simulink model "Simulacion_stepper_2024a"  (R2024a)
settings: Solver=ode4  StartTime=0.0  StopTime=Time_simulation  FixedStep=1/frecuency_simulation  RelTol=1e-3
InitFcn:
  | %%InitFcn();
StopFcn:
  | %%FinishFcn
model workspace (MAT data in the model file):
  Ts_stepper = 0.001
values from neighbouring files (symbols this model uses):
  B = motor_params.B_internal    [bode.m]    (also in current_observer.m = 0.0005; discretizacion.m = [ 1/L, 0; ekf_4_estados.m = params.B; obs_ctrl_back_emf_ext.m = [1/L 0)
  B0 = 3*wn_w - BJ_hat    [Barrido_B.m]    (also in Barrido_J.m; InitFcn.m = 449.962302294)
  B1 = 3*wn_w^2 - B0*BJ_hat    [Barrido_B.m]    (also in Barrido_J.m; InitFcn.m = 64448.3670019)
  B2 = -(J_var/P)*(wn_w^3)    [Barrido_B.m]    (also in Barrido_J.m; InitFcn.m = -0.364323750994)
  B_internal = 1e-4    (= 0.0001)    [InitFcn.m]
  B_var = B_internal* B_factors(k)    [Barrido_B.m]    (also in Barrido_J.m = B_real; InitFcn.m = 0.0001)
  frecuency_simulation = 10e3    (= 10000)    [InitFcn.m]
  I_nom = 1    [InitFcn.m]    (also in salient_motor.m)
  J = motor_params.J_internal    [bode.m]    (also in current_observer.m = 0.008; ekf_4_estados.m = params.J; obs_ctrl_back_emf_ext.m = 0.008; obs_y_contrl_back_emd.m = 0.008)
  J_internal = 4.7/1000000    (= 4.7e-06)    [InitFcn.m]
  J_var = J_real    [Barrido_B.m]    (also in Barrido_J.m = J_internal * J_factors(k); InitFcn.m = 4.7e-06)
  Ke = Kt    [InitFcn.m]    (also in current_observer.m = 0.0055; ekf_4_estados.m = params.Ke; observer.m = Pvec(3); salient_motor.m = 0.0066)
  Ki_d = wd_d*R    (= 3926.99081699)    [InitFcn.m]    (also in bode.m = PI_dq_params.Ki_d_salient)
  Ki_d_salient = wd_d^2*Ld    (= 21491.0635834)    [InitFcn.m]
  Ki_q = wd_q*R    (= 3926.99081699)    [InitFcn.m]    (also in bode.m = PI_dq_params.Ki_q_salient)
  Ki_q_salient = wd_q^2*Lq    (= 7846.33549887)    [InitFcn.m]
  Ki_w = (wn_w^2)*J_var/Kt    [Barrido_B.m]    (also in Barrido_J.m; InitFcn.m; bode.m = PI_MTPA_params.Ki_w)
  Kp_d = wd_d*L    (= 9.42477796077)    [InitFcn.m]    (also in bode.m = PI_dq_params.Kp_d_salient)
  Kp_d_salient = 2*shi_d*wd_d*Ld -R    (= 16.845833313)    [InitFcn.m]
  Kp_q = wd_q*L    (= 9.42477796077)    [InitFcn.m]    (also in bode.m = PI_dq_params.Kp_q_salient)
  Kp_q_salient = 2*shi_q*wd_q*Lq-R    (= 4.56311709936)    [InitFcn.m]
  Kp_w = (2*shi_w*wn_w*J_var)/Kt    [Barrido_B.m]    (also in Barrido_J.m; InitFcn.m; bode.m = PI_MTPA_params.Kp_w)
  Kt = Thold / (sqrt(2) * I_nom)    [InitFcn.m]    (also in current_observer.m = 0.275; ekf_4_estados.m = params.Kt; frecuencia_max.m = 0.33; observer.m = Pvec(4))
  L = 6/1000    (= 0.006)    [InitFcn.m]    (also in current_observer.m = place(A', C', 10*eig(A)).'; desfase.m = lags(k); discretizacion.m = 0.01; frecuencia_max.m)
  Ld = L0 + L2    [Copy_of_PMSM_salient.m]    (also in InitFcn.m = 0.00871; bode.m = motor_params.Ld; ekf_4_estados.m = params.Ld; salient_motor.m = 0.00871)
  Lq = L0 - L2    [Copy_of_PMSM_salient.m]    (also in InitFcn.m = 0.00318; bode.m = motor_params.Lq; ekf_4_estados.m = params.Lq; salient_motor.m = 0.00318)
  N_steps = 360/Step_angle    (= 200)    [InitFcn.m]
  P = N_teeths/2    (= 50)    [InitFcn.m]    (also in bode.m = motor_params.P; ekf_4_estados.m = P_pred; frecuencia_max.m; salient_motor.m)
  Phi = pi/2    (= 1.57079632679)    [InitFcn.m]    (also in ekf_4_estados.m = eye(4) + Ts_eff*A)
  Psi = Kt/P    [InitFcn.m]    (also in bode.m = motor_params.Ke; salient_motor.m = 0.0066)
  R = 2.5    [InitFcn.m]    (also in bode.m = motor_params.R; current_observer.m = 3.4; discretizacion.m = 3.4; ekf_4_estados.m = params.R)
  sample_time = 1/frecuency_simulation    (= 0.0001)    [InitFcn.m]
  Tdm = 18/1000    (= 0.018)    [InitFcn.m]    (also in salient_motor.m)
  Ts_current = 1/f_current    (= 0.0001)    [InitFcn.m]
  Ts_DO = Ts_Wm    (= 0.0001)    [InitFcn.m]
  Ts_ekf = 1/f_ekf    (= 0.0001)    [InitFcn.m]
  Ts_Wm = Ts_current    (= 0.0001)    [InitFcn.m]
  Vdc = 12    [InitFcn.m]    (also in frecuencia_max.m)
undefined symbols (not defined in the file or in its folder): DiscIntNeverNeededParam
libraries: fl_lib x27, nesl_utility x19, spsMosfetLib x16, simulink x8, eeTransforms x4, spsDCVoltageSourceLib x4, spsVoltageMeasurementLib x4, ee_lib x3, slexportprevious_tp74def212_4eb8_4616_a2bc_f4e795655e99 x1, spsTriangleGeneratorLib x1, spspowerguiLib x1
(part 1 of 4)
settings Model: DataTypeOverride=Off  SimulationMode=accelerator  Creator=PC  LastModifiedBy=damia
settings DataIOCC: Decimation=20  ReturnWorkspaceOutputs=off
settings OptimizationCC: OptimizeBlockIOStorage=off  OptimizeDataStoreBuffers=off  BusAssignmentInplaceUpdate=off  UseRowMajorAlgorithm=on
settings DebuggingCC: SFUnexpectedBacktrackingDiag=warning  SFNoUnconditionalDefaultTransitionDiag=warning
settings RTWCC: GenerateReport=on  BuildConfiguration=Debug  LaunchReport=on
settings CodeAppCC: ForceParamTrailComments=on  MATLABSourceComments=on  EnableCustomComments=on
settings GRTTargetCC: CombineSignalStateStructs=on  SupportVariableSizeSignals=on  MultiInstanceErrorCode=Warning
settings ConfigComp: CovBoundaryAbsTol=1.0e-5
settings SimscapeCC: ExplicitSolverDiagnosticOptions=none

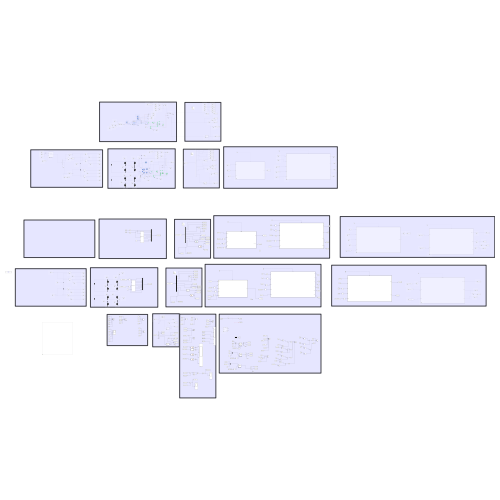
[thumbnail: Simulink's stored preview of the top-level diagram]
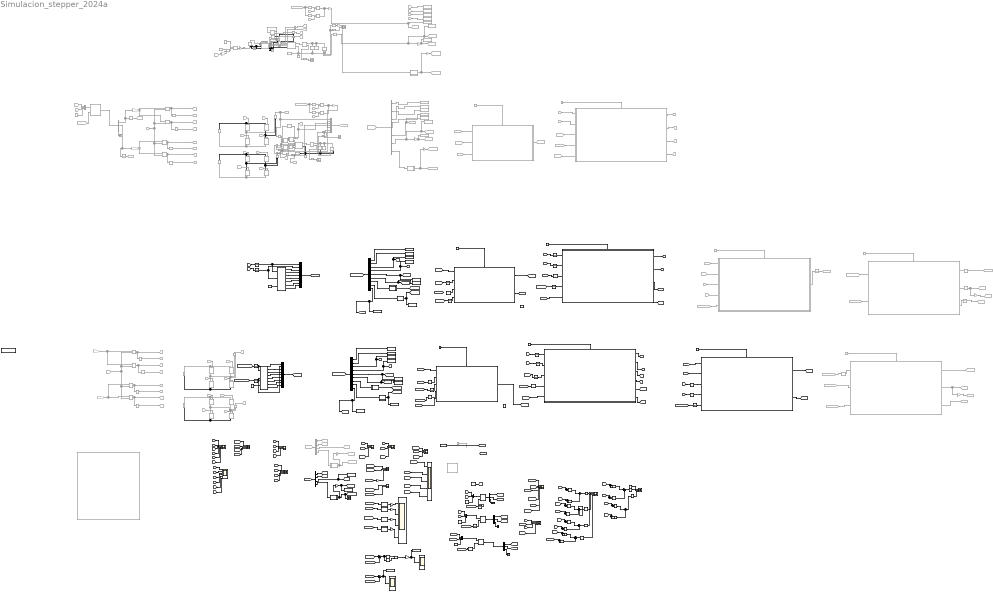
== system Simulacion_stepper_2024a ==
  note: A
  note: A
  note: Vab
      | Iab,
      | Te(N*m),
      | We(rad/s),
      | Theta_e(rad)
  note: A
  note: A
  note: A
  note: Vab
      | Iab,
      | Te(N*m),
      | We(rad/s),
      | Theta_e(rad)
  note: A
  note: Vab
      | Iab,
      | Te(N*m),
      | We(rad/s),
      | Theta_e(rad)
  note: Vab
      | Iab,
      | Te(N*m),
      | We(rad/s),
      | Theta_e(rad)
  1/step angle : Gain  Commented=on  Gain=1/1.8  SaturateOnIntegerOverflow=on  OutDataTypeStr=Inherit: Same as input  ParamDataTypeStr=Inherit: Same as input
  Atan2 : Trigonometry  Operator=atan2
  Clarke to Park Angle Transform : eeTransforms/Clarke to Park Angle Transform  AxisAlignment=D-axis
      settings: LibrarySourceBlock=|
      | ee_sl_lib/Mathematical
      | Transforms/Clarke to Park
      | Angle Transform
  Clarke to Park Angle Transform1 : eeTransforms/Clarke to Park Angle Transform  AxisAlignment=D-axis
      settings: LibrarySourceBlock=|
      | ee_sl_lib/Mathematical
      | Transforms/Clarke to Park
      | Angle Transform
  Constant : Constant  Value=0.2
  Constant1 : Constant  Value=Vdc
  Constant10 : Constant  Commented=on  Value=0  OutDataTypeStr=double
  Constant11 : Constant  Value=0  OutDataTypeStr=double
  Constant2 : Constant  Value=0  OutDataTypeStr=double
  Constant3 : Constant  Value=0.2
  Constant4 : Constant  Commented=on  Value=0.5
  Constant5 : Constant  Commented=on  Value=2*pi
  Constant6 : Constant  Value=0  OutDataTypeStr=double
  Constant7 : Constant  Value=0
  Constant8 : Constant  Value=0
  Controlled Voltage Source : fl_lib/Electrical/Electrical Sources/Controlled Voltage Source  Commented=on
  Controlled Voltage Source1 : fl_lib/Electrical/Electrical Sources/Controlled Voltage Source  Commented=on
  Controlled Voltage Source2 : fl_lib/Electrical/Electrical Sources/Controlled Voltage Source  Commented=on
  Cos : Trigonometry  Commented=on  Operator=cos
  Cos1 : Trigonometry  Commented=on  Operator=cos
  Cos3 : Trigonometry  Operator=cos
  Current Sensor{,1..3} (4 alike) : fl_lib/Electrical/Electrical Sensors/Current Sensor  Commented=on
  DC Voltage Source{1..4} (4 alike) : spsDCVoltageSourceLib/DC Voltage Source  Commented=on  Amplitude=Vdc  Measurements=None
  Demux : Demux  Outputs=9
  Demux1 : Demux  Outputs=3
  Demux2 : Demux  Outputs=3
  Demux3 : Demux  Commented=on  Outputs=7
  Demux4 : Demux  Commented=on  Outputs=3
  Demux5 : Demux  Outputs=3
  Demux6 : Demux  Outputs=9
  Divide : Product  Commented=on  Inputs=*/
  ENA or step rate : Scope  Commented=on
  ERef A+ : fl_lib/Electrical/Electrical Elements/Electrical Reference  Commented=on
  ERef B-{,1..3} (4 alike) : fl_lib/Electrical/Electrical Elements/Electrical Reference  Commented=on
  From : From  Commented=on  GotoTag=Wm_ref
  From103 : From  Commented=on  GotoTag=Vb_M0
  From104 : From  Commented=on  GotoTag=S1_M1
  From105 : From  Commented=on  GotoTag=Vd_M1
  From106 : From  Commented=on  GotoTag=Vq_M1
  From107 : From  Commented=on  GotoTag=S3_M1
  From108 : From  Commented=on  GotoTag=theta_e_planta_M1  TagVisibility=global
  From109 : From  Commented=on  GotoTag=S2_M1
  From11 : From  Commented=on  GotoTag=S4_M2
  From110 : From  Commented=on  GotoTag=Ib_M0
  From111 : From  Commented=on  GotoTag=S4_M1
  From112 : From  Commented=on  GotoTag=Ia_M0
  From115 : From  Commented=on  GotoTag=S5_M1
  From116 : From  Commented=on  GotoTag=S7_M1
  From117 : From  Commented=on  GotoTag=S6_M1
  From118 : From  Commented=on  GotoTag=carrier
  From128 : From  Commented=on  GotoTag=Valpha_M2
  From129 : From  Commented=on  GotoTag=Vbetha_M2
  From130 : From  Commented=on  GotoTag=Ia_M2
  From131 : From  Commented=on  GotoTag=Ib_M2
  From132 : From  Commented=on  GotoTag=Iq_obs_M2
  From136 : From  Commented=on  GotoTag=theta_e_planta_M2  TagVisibility=global
  From159 : From  Commented=on  GotoTag=theta_e_planta_M2  TagVisibility=global
  From19 : From  Commented=on  GotoTag=x_ekf_4var_M1
  From24 : From  Commented=on  GotoTag=Iq_obs_M2
  From3 : From  Commented=on  GotoTag=Id_obs_M2
  From38 : From  Commented=on  GotoTag=theta_e_planta_M1  TagVisibility=global
  From39 : From  Commented=on  GotoTag=S5_M2
  From4 : From  Commented=on  GotoTag=S1_M2
  From40 : From  Commented=on  GotoTag=S7_M2
  From48 : From  Commented=on  GotoTag=S6_M2
  From59 : From  Commented=on  GotoTag=carrier
  From62 : From  Commented=on  GotoTag=S8_M2
  From63 : From  Commented=on  GotoTag=Ia_M1
  From65 : From  Commented=on  GotoTag=Wm_ref
  From69 : From  Commented=on  GotoTag=theta_e_planta_M2  TagVisibility=global
  From7 : From  Commented=on  GotoTag=S3_M2
  From85 : From  Commented=on  GotoTag=Wm_planta_M1  TagVisibility=global
  From86 : From  Commented=on  GotoTag=Ib_M1
  From87 : From  Commented=on  GotoTag=theta_e_planta_M1  TagVisibility=global
  From88 : From  Commented=on  GotoTag=Wm_planta_M1  TagVisibility=global
  From89 : From  Commented=on  GotoTag=var_stepper_M1
  From9 : From  Commented=on  GotoTag=S2_M2
  From90 : From  Commented=on  GotoTag=Ia_M1
  From91 : From  Commented=on  GotoTag=Iq_ref_M1  TagVisibility=global
  From92 : From  Commented=on  GotoTag=Tx_hat_M1
  From93 : From  Commented=on  GotoTag=Ib_M1
  From94 : From  Commented=on  GotoTag=theta_e_planta_M0  TagVisibility=global
  From95 : From  Commented=on  GotoTag=Ia_M0
  From96 : From  Commented=on  GotoTag=Ib_M0
  From97 : From  Commented=on  GotoTag=S8_M1
  From98 : From  Commented=on  GotoTag=Va_M0
  Function-Call Generator : slexportprevious_tp74def212_4eb8_4616_a2bc_f4e795655e99/Function-Call Generator  sample_time=Ts_ekf  numberOfIterations=1  DisallowWideOutput=off
  Function-Call Generator1 : FunctionCallGenerator  Commented=on  SampleTime=Ts_ekf
  Function-Call Generator10 : FunctionCallGenerator  Commented=on  SampleTime=1/1000
  Function-Call Generator2 : FunctionCallGenerator  Commented=on  SampleTime=Ts_DO
  Function-Call Generator3 : FunctionCallGenerator  Commented=on  SampleTime=Ts_DO
  Function-Call Generator4 : FunctionCallGenerator  SampleTime=Ts_current
  Function-Call Generator5 : FunctionCallGenerator  SampleTime=Ts_Wm
  Function-Call Generator6 : FunctionCallGenerator  Commented=on  SampleTime=Ts_current
  Function-Call Generator7 : FunctionCallGenerator  Commented=on  SampleTime=Ts_Wm
  Function-Call Generator8 : FunctionCallGenerator  SampleTime=Ts_current
  Function-Call Generator9 : FunctionCallGenerator  SampleTime=Ts_Wm
  Gain : Gain  Commented=on  Gain=200
  Gain{1,8..9,13} (4 alike) : Gain  Commented=on  Gain=2/Vdc  OutDataTypeStr=double
  Gain10 : Gain  Commented=on  Gain=5
  Gain{7,11..12,14..15} (5 alike) : Gain  Commented=on  Gain=P  OutDataTypeStr=double
  Gain17 : Gain  Commented=on  Gain=Kt
  Gain18 : Gain  Commented=on  Gain=Kt
  Gain20 : Gain
  Gain{21,25..26,28,30} (5 alike) : Gain  Gain=180/pi
  Gain3 : Gain  Commented=on  Gain=1/P
  Gain4 : Gain  Gain=P  OutDataTypeStr=double
  Gain5 : Gain  Commented=on  Gain=1/P
  Goto1 : Goto  Commented=on  GotoTag=S1_M2
  Goto100 : Goto  Commented=on  GotoTag=We_hat_M2
  Goto101 : Goto  Commented=on  GotoTag=Tx_hat_M2
  Goto104 : Goto  Commented=on  GotoTag=theta_e_hat_M2
  Goto105 : Goto  Commented=on  GotoTag=Wm_hat_M2
  Goto13 : Goto  Commented=on  GotoTag=S3_M2
  Goto14 : Goto  Commented=on  GotoTag=Ib_M0
  Goto15 : Goto  Commented=on  GotoTag=Vb_M0
  Goto16 : Goto  Commented=on  GotoTag=Va_M0
  Goto17 : Goto  Commented=on  GotoTag=Va_M2
  Goto18 : Goto  Commented=on  GotoTag=S4_M2
  Goto2 : Goto  Commented=on  GotoTag=S2_M2
  Goto22 : Goto  Commented=on  GotoTag=S5_M2
  Goto23 : Goto  Commented=on  GotoTag=S6_M2
  Goto25 : Goto  Commented=on  GotoTag=S7_M2
  Goto26 : Goto  Commented=on  GotoTag=S1_M1
  Goto28 : Goto  Commented=on  GotoTag=Ia_obs_M1
  Goto29 : Goto  Commented=on  GotoTag=Ib_obs_M1
  Goto30 : Goto  Commented=on  GotoTag=Wm_obs_M1
  Goto31 : Goto  Commented=on  GotoTag=theta_m_obs_M1
  Goto32 : Goto  Commented=on  GotoTag=S2_M1
  Goto33 : Goto  Commented=on  GotoTag=S8_M2
  Goto34 : Goto  Commented=on  GotoTag=We_hat_M2
  Goto35 : Goto  Commented=on  GotoTag=Tx_hat_M2
  Goto4 : Goto  Commented=on  GotoTag=Ia_M0
  Goto42 : Goto  Commented=on  GotoTag=theta_e_obs_M1
  Goto44 : Goto  Commented=on  GotoTag=theta_e_hat_M2
  Goto45 : Goto  Commented=on  GotoTag=Wm_hat_M2
  Goto48 : Goto  Commented=on  GotoTag=var_stepper_M1
  Goto50 : Goto  Commented=on  GotoTag=Vd_M1
  Goto51 : Goto  Commented=on  GotoTag=Vb_M2
  Goto54 : Goto  Commented=on  GotoTag=Vq_M1
  Goto56 : Goto  Commented=on  GotoTag=Ia_M1
  Goto57 : Goto  Commented=on  GotoTag=Ib_M1
  Goto58 : Goto  Commented=on  GotoTag=Wm_planta_M1  TagVisibility=global
  Goto59 : Goto  Commented=on  GotoTag=We_planta_M1  TagVisibility=global
  Goto60 : Goto  Commented=on  GotoTag=theta_e_planta_M1  TagVisibility=global
  Goto61 : Goto  Commented=on  GotoTag=theta_m_planta_M1
  Goto62 : Goto  Commented=on  GotoTag=Te_planta_M1  TagVisibility=global
  Goto63 : Goto  Commented=on  GotoTag=S3_M1
  Goto67 : Goto  Commented=on  GotoTag=Id_M1
  Goto69 : Goto  Commented=on  GotoTag=Iq_ref_M1  TagVisibility=global
  Goto70 : Goto  Commented=on  GotoTag=S4_M1
  Goto71 : Goto  Commented=on  GotoTag=Valpha_M1
  Goto72 : Goto  Commented=on  GotoTag=Vbetha_M1
  Goto73 : Goto  Commented=on  GotoTag=S5_M1
  Goto75 : Goto  Commented=on  GotoTag=S6_M1
  Goto76 : Goto  Commented=on  GotoTag=S7_M1
  Goto77 : Goto  Commented=on  GotoTag=S8_M1
  Goto78 : Goto  Commented=on  GotoTag=Va_M1
  Goto79 : Goto  Commented=on  GotoTag=Vb_M1
  Goto80 : Goto  Commented=on  GotoTag=Iq_M1
  Goto88 : Goto  Commented=on  GotoTag=Wm_planta_M0  TagVisibility=global
  Goto89 : Goto  Commented=on  GotoTag=We_planta_M0  TagVisibility=global
  Goto90 : Goto  Commented=on  GotoTag=theta_e_planta_M0  TagVisibility=global
  Goto91 : Goto  Commented=on  GotoTag=theta_m_planta_M0
  Goto92 : Goto  Commented=on  GotoTag=Te_planta_M0  TagVisibility=global
  Goto97 : Goto  Commented=on  GotoTag=x_ekf_4var_M2
  Iab : Scope  NumInputPorts=6
  Id : Scope  NumInputPorts=4
  Ideal Rotational Motion Sensor : fl_lib/Mechanical/Mechanical Sensors/Ideal Rotational Motion Sensor  Commented=on  reference=foundation.enum.MeasurementReference.difference  acceleration_port=false  velocity_port=true  position_port=true  wrap_angle=false  offset=0 rad
  Ideal Rotational Motion Sensor1 : fl_lib/Mechanical/Mechanical Sensors/Ideal Rotational Motion Sensor  Commented=on  reference=foundation.enum.MeasurementReference.difference  acceleration_port=false  velocity_port=true  position_port=true  wrap_angle=false  offset=0 rad
  Ideal Torque Sensor : fl_lib/Mechanical/Mechanical Sensors/Ideal Torque Sensor  Commented=on
  Ideal Torque Sensor1 : fl_lib/Mechanical/Mechanical Sensors/Ideal Torque Sensor  Commented=on
  Idq : Scope  NumInputPorts=4
  Imag : Scope  NumInputPorts=4
  Inertia : fl_lib/Mechanical/Rotational Elements/Inertia  Commented=on  inertia=J_external kg*m^2  num_ports=foundation.enum.numPorts2.one  w_specify=on  w_priority=Low  w="InitialSpeed  rad/s"  w_nominal_specify=off  w_nominal_value=1  w_nominal_unit=rad/s  t_specify=off  t_priority=None  t=0 N*m  t_nominal_specify=off  t_nominal_value=1  t_nominal_unit=N*m
  Inertia1 : fl_lib/Mechanical/Rotational Elements/Inertia  Commented=on  inertia=J_external kg*m^2  num_ports=foundation.enum.numPorts2.one  w_specify=on  w_priority=Low  w="InitialSpeed  rad/s"  w_nominal_specify=off  w_nominal_value=1  w_nominal_unit=rad/s  t_specify=off  t_priority=None  t=0 N*m  t_nominal_specify=off  t_nominal_value=1  t_nominal_unit=N*m
  Iq : Scope  NumInputPorts=6
  Level-2 MATLAB S-Function : M-S-Function  FunctionName=PMSM_salient  Parameters=params
  Level-2 MATLAB S-Function1 : M-S-Function  FunctionName=PMSM_salient_dq  Parameters=params
  MATLAB Function1 : MATLAB Function  TreatAsAtomicUnit=on
  MATLAB Function10 : MATLAB Function  TreatAsAtomicUnit=on
  MATLAB Function11 : MATLAB Function  TreatAsAtomicUnit=on
  MATLAB Function12 : MATLAB Function  TreatAsAtomicUnit=on
  MATLAB Function14 : MATLAB Function  TreatAsAtomicUnit=on
  MATLAB Function2 : MATLAB Function  Commented=on  TreatAsAtomicUnit=on
  MATLAB Function3 : MATLAB Function  TreatAsAtomicUnit=on
  MATLAB Function4 : MATLAB Function  TreatAsAtomicUnit=on
  MATLAB Function5 : MATLAB Function  Commented=on  TreatAsAtomicUnit=on
  MATLAB Function6 : MATLAB Function  Commented=on  TreatAsAtomicUnit=on
  MATLAB Function8 : MATLAB Function  TreatAsAtomicUnit=on
  MATLAB Function9 : MATLAB Function  TreatAsAtomicUnit=on
  MRRef Motor : fl_lib/Mechanical/Rotational Elements/Mechanical Rotational Reference  Commented=on
  MRRef Motor2 : fl_lib/Mechanical/Rotational Elements/Mechanical Rotational Reference  Commented=on
  Meas 1 : Subsystem  Commented=on
      mask Display: disp('v')
  Mosfet{1..16} (16 alike) : spsMosfetLib/Mosfet  Commented=on  Ron=0.1  Lon=0  Rd=0.01  Vfd=0  IC=0  Rs=1e5  Cs=inf  Measurements=on
  Mux : Mux  Commented=on  Inputs=7
  Mux1 : Mux  Commented=on  Inputs=3
  Mux2 : Mux  Inputs=3
  Mux3 : Mux  Inputs=3
  Mux4 : Mux  Inputs=9
  Mux5 : Mux  Inputs=3
  Mux6 : Mux  Inputs=9
  NOT{1..8} (8 alike) : Logic  Commented=on  Operator=NOT  IconShape=distinctive  AllPortsSameDT=off  OutDataTypeStr=boolean
  PS-Simulink Converter : nesl_utility/PS-Simulink Converter  Commented=on  PhysicalDomain=network_engine_domain  SubClassName=ps_output  LeftPortType=input  RightPortType=output  PseudoPeriodic=off  Frequencies=[]  VectorFormat=inherit  Unit=V  AffineConversion=off
  PS-Simulink Converter1 : nesl_utility/PS-Simulink Converter  Commented=on  PhysicalDomain=network_engine_domain  SubClassName=ps_output  LeftPortType=input  RightPortType=output  PseudoPeriodic=off  Frequencies=[]  VectorFormat=inherit  Unit=V  AffineConversion=off
  PS-Simulink Converter2 : nesl_utility/PS-Simulink Converter  Commented=on  PhysicalDomain=network_engine_domain  SubClassName=ps_output  LeftPortType=input  RightPortType=output  PseudoPeriodic=off  Frequencies=[]  VectorFormat=inherit  Unit=A  AffineConversion=off
  PS-Simulink Converter3 : nesl_utility/PS-Simulink Converter  Commented=on  PhysicalDomain=network_engine_domain  SubClassName=ps_output  LeftPortType=input  RightPortType=output  PseudoPeriodic=off  Frequencies=[]  VectorFormat=inherit  Unit=A  AffineConversion=off
  PS-Simulink Converter4 : nesl_utility/PS-Simulink Converter  Commented=on  PhysicalDomain=network_engine_domain  SubClassName=ps_output  LeftPortType=input  RightPortType=output  PseudoPeriodic=off  Frequencies=[]  VectorFormat=inherit  Unit=inherit  AffineConversion=off
  PS-Simulink Converter5 : nesl_utility/PS-Simulink Converter  Commented=on  PhysicalDomain=network_engine_domain  SubClassName=ps_output  LeftPortType=input  RightPortType=output  PseudoPeriodic=off  Frequencies=[]  VectorFormat=inherit  Unit=inherit  AffineConversion=off
  PS-Simulink Converter6 : nesl_utility/PS-Simulink Converter  Commented=on  PhysicalDomain=network_engine_domain  SubClassName=ps_output  LeftPortType=input  RightPortType=output  PseudoPeriodic=off  Frequencies=[]  VectorFormat=inherit  Unit=rad/s  AffineConversion=off
  PS-Simulink Converter7 : nesl_utility/PS-Simulink Converter  Commented=on  PhysicalDomain=network_engine_domain  SubClassName=ps_output  LeftPortType=input  RightPortType=output  PseudoPeriodic=off  Frequencies=[]  VectorFormat=inherit  Unit=inherit  AffineConversion=off
  Park to Clarke Angle Transform : eeTransforms/Park to Clarke Angle Transform  AxisAlignment=Q-axis
      settings: LibrarySourceBlock=|
      | ee_sl_lib/Mathematical
      | Transforms/Park to Clarke
      | Angle Transform
  Park to Clarke Angle Transform1 : eeTransforms/Park to Clarke Angle Transform  Commented=on  AxisAlignment=D-axis
      settings: LibrarySourceBlock=|
      | ee_sl_lib/Mathematical
      | Transforms/Park to Clarke
      | Angle Transform
  Product{,1..7,14..17} (12 alike) : Product
  Product{8..11} (4 alike) : Product  Commented=on
  Relational Operator{1..4} (4 alike) : RelationalOperator  Commented=on  OutDataTypeStr=fixdt(1,16)  RndMeth=Simplest  InputSameDT=off
  Relational Operator{5..8} (4 alike) : RelationalOperator  Commented=on  Operator=<  OutDataTypeStr=fixdt(1,16)  RndMeth=Simplest  InputSameDT=off
  Results : Scope  Commented=on  NumInputPorts=2
  Rotational Friction1 : fl_lib/Mechanical/Rotational Elements/Rotational Friction  Commented=on  brkwy_trq=Tba N*m  brkwy_vel=Wba rad/s  Col_trq=Tc N*m  visc_coef=B_external N*m*s/rad  w_specify=off  w_priority=None  w=0 rad/s  w_nominal_specify=off  w_nominal_value=1  w_nominal_unit=rad/s  t_specify=off  t_priority=None  t=0 N*m  t_nominal_specify=off  t_nominal_value=1  t_nominal_unit=N*m
  Rotational Friction3 : fl_lib/Mechanical/Rotational Elements/Rotational Friction  Commented=on  brkwy_trq=Tba N*m  brkwy_vel=Wba rad/s  Col_trq=Tc N*m  visc_coef=B_external N*m*s/rad  w_specify=off  w_priority=None  w=0 rad/s  w_nominal_specify=off  w_nominal_value=1  w_nominal_unit=rad/s  t_specify=off  t_priority=None  t=0 N*m  t_nominal_specify=off  t_nominal_value=1  t_nominal_unit=N*m
  Scope : Scope  Commented=on
  Scope1 : Scope  Commented=on
  Scope12 : Scope  NumInputPorts=3
  Scope14 : Scope
  Scope15 : Scope
  Scope2 : Scope  NumInputPorts=5
  Scope24 : Scope  Commented=on
  Scope4 : Scope
  Scope5 : Scope  NumInputPorts=2
  Scope6 : Scope  NumInputPorts=3
  Simulink-PS Converter : nesl_utility/Simulink-PS Converter  Commented=on  PhysicalDomain=network_engine_domain  SubClassName=ps_input  LeftPortType=input  RightPortType=output  PseudoPeriodic=off  Frequencies=[]  NoiseDistribution=none  NoiseParameters=[]  Unit=1  AffineConversion=off  FilteringAndDerivatives=provide  SimscapeFilterOrder=1  InputFilterTimeConstant=0.001  UdotUserProvided=0
  Simulink-PS Converter1 : nesl_utility/Simulink-PS Converter  Commented=on  PhysicalDomain=network_engine_domain  SubClassName=ps_input  LeftPortType=input  RightPortType=output  PseudoPeriodic=off  Frequencies=[]  NoiseDistribution=none  NoiseParameters=[]  Unit=1  AffineConversion=off  FilteringAndDerivatives=provide  SimscapeFilterOrder=1  InputFilterTimeConstant=0.001  UdotUserProvided=0
  Simulink-PS Converter2 : nesl_utility/Simulink-PS Converter  Commented=on  PhysicalDomain=network_engine_domain  SubClassName=ps_input  LeftPortType=input  RightPortType=output  PseudoPeriodic=off  Frequencies=[]  NoiseDistribution=none  NoiseParameters=[]  Unit=1  AffineConversion=off  FilteringAndDerivatives=provide  SimscapeFilterOrder=1  InputFilterTimeConstant=0.001  UdotUserProvided=0
  Sin : Trigonometry  Commented=on
  Sin1 : Trigonometry  Commented=on
  Sin3 : Trigonometry
  Solver Configuration : nesl_utility/Solver Configuration  Commented=on  PhysicalDomain=network_engine_domain  SubClassName=solver  LeftPortType=input  RightPortType=generic  Tones=[]  Harmonics=[]  SimulateNoise=off  Profile=off  UseLocalSampling=off  EnableSwitchedLinearOptims=on  FrequencyDomain=off  UseCCode=off  RelTol=0.001  AbsTol=1e-06  MinStep=1e-09  ToWorkspace=off  RevertToSquareIcSolve=off  NumHomotopyIterations=100  PhasorMode=off  PhasorModeNumHarmonics=1  ConsistencySolver=NEWTON_FTOL  IndexReductionMethod=DerivativeReplacement  DoDC=off  ResidualTolerance=1e-9  ConsistencyTolSource=GLOBAL  ConsistencyAbsTol=0.001  ConsistencyRelTol=0.001  ConsistencyTolFactor=0.001  UseLocalSolver=on  LocalSolverChoice=NE_BACKWARD_EULER_ADVANCER  ResolveIndetEquations=on  FunctionEvalNumThread=1  LocalSolverSampleTime=1/frecuency_simulation  DoFixedCost=on  MaxNonlinIter=3  MaxModeIter=2  ComputeImpulses=off  ImpulseIterations=2  LinearAlgebra=auto  LinearAlgebraNumThread=0  EquationFormulation=NE_TIME_EF  DelaysMemoryBudget=1024  AutomaticFiltering=on  FilteringTimeConstant=0.001  PartitionStorageMethod=AS_NEEDED  PartitionMemoryBudget=1024  PartitionMethod=FAST  MultibodyUseLocalSolver=off  MultibodyLocalSolverChoice=ODE1  MultibodyLocalSolverSampleTime=0.001
  Solver Configuration1 : nesl_utility/Solver Configuration  Commented=on  PhysicalDomain=network_engine_domain  SubClassName=solver  LeftPortType=input  RightPortType=generic  Tones=[]  Harmonics=[]  SimulateNoise=off  Profile=off  UseLocalSampling=off  EnableSwitchedLinearOptims=on  FrequencyDomain=off  UseCCode=off  RelTol=0.001  AbsTol=1e-06  MinStep=1e-09  ToWorkspace=off  RevertToSquareIcSolve=off  NumHomotopyIterations=100  PhasorMode=off  PhasorModeNumHarmonics=1  ConsistencySolver=NEWTON_FTOL  IndexReductionMethod=DerivativeReplacement  DoDC=off  ResidualTolerance=1e-9  ConsistencyTolSource=GLOBAL  ConsistencyAbsTol=0.001  ConsistencyRelTol=0.001  ConsistencyTolFactor=0.001  UseLocalSolver=on  LocalSolverChoice=NE_BACKWARD_EULER_ADVANCER  ResolveIndetEquations=on  FunctionEvalNumThread=1  LocalSolverSampleTime=1/frecuency_simulation  DoFixedCost=on  MaxNonlinIter=3  MaxModeIter=2  ComputeImpulses=off  ImpulseIterations=2  LinearAlgebra=auto  LinearAlgebraNumThread=0  EquationFormulation=NE_TIME_EF  DelaysMemoryBudget=1024  AutomaticFiltering=on  FilteringTimeConstant=0.001  PartitionStorageMethod=AS_NEEDED  PartitionMemoryBudget=1024  PartitionMethod=FAST  MultibodyUseLocalSolver=off  MultibodyLocalSolverChoice=ODE1  MultibodyLocalSolverSampleTime=0.001
  Sqrt{,1..5} (6 alike) : Sqrt
  Stepper Motor : ee_lib/Electromechanical/Reluctance & Stepper/Stepper Motor  Commented=on  step_or_av=1  Ra=R Ohm  La=L H  Km=Kt N*m/A  Td=Tdm m*mN  Rm=Inf Ohm  w_vec=[ 0 200 1000 ] rpm  T_vec=[ 2.2 2.2 1 ] N*m  assert_if_slipping=1  J_total=J+1e-3 kg*m^2  max_step_rate=max_step_rate Hz  Step=1.8 deg  J=J_internal kg*m^2  B=B_internal N*m/(rad/s)  speed0=InitialSpeed rad/s  theta0=0 deg  alpha=[.00393, .00393] 1/K  Tmeas=25 degC  Tmeas2=125 degC  T_vec2=[1.7, 1.7, .85] N*m  half_stepping=ee.enum.electromech.steppingModeAveraged.fullStep  thermal_masses=[100, 100] J/K  initial_temperatures=[25, 25] degC  rotor_thermal_mass=50 J/K  rotor_initial_temperature=25 degC  Rm_percent_rotor=90
      settings: InternalSimscapePortConfiguration="{\"Bottom\":[],\"Left\":[{\"id\":\"pA\",\"label\":\"A+\",\"type\":\"foundation.electrical.electrical\"},{\"id\":\"nA\",\"label\":\"A-\",\"type\":\"foundation.electrical.electrical\"},{\"id\":\"pB\",\"label\":\"B+\",\"type\":\"foundation.electrical.electrical\"},{\"id\":\"nB\",\"label\":\"B-\",\"type\":\"foundation.electrical.electrical\"}],\"Right\":[{\"id\":\"R\",\"label\":\"R\",\"type\":\"foundation.mechanical.rotational.rotational\"},{\"id\":\"C\",\"label\":\"C\",\"type\":\"foundation.mechanical.rotational.rotational\"}],\"Top\":[]}"
  Stepper Motor1 : ee_lib/Electromechanical/Reluctance & Stepper/Stepper Motor  Commented=on  step_or_av=ee.enum.electromech.simulationMode.stepping  Ra=R Ohm  La=L H  Km=Kt N*m/A  Td=Tdm m*mN  Rm=Inf Ohm  w_vec=[ 0 200 1000 ] rpm  T_vec=[ 2.2 2.2 1 ] N*m  assert_if_slipping=1  J_total=J+1e-3 kg*m^2  max_step_rate=max_step_rate Hz  Step=1.8 deg  J=J_internal kg*m^2  B=B_internal N*m/(rad/s)  speed0=InitialSpeed rad/s  theta0=0 deg  alpha=[.00393, .00393] 1/K  Tmeas=25 degC  Tmeas2=125 degC  T_vec2=[1.7, 1.7, .85] N*m  half_stepping=ee.enum.electromech.steppingModeAveraged.fullStep  thermal_masses=[100, 100] J/K  initial_temperatures=[25, 25] degC  rotor_thermal_mass=50 J/K  rotor_initial_temperature=25 degC  Rm_percent_rotor=90
      settings: InternalSimscapePortConfiguration="{\"Bottom\":[],\"Left\":[{\"id\":\"pA\",\"label\":\"A+\",\"type\":\"foundation.electrical.electrical\"},{\"id\":\"nA\",\"label\":\"A-\",\"type\":\"foundation.electrical.electrical\"},{\"id\":\"pB\",\"label\":\"B+\",\"type\":\"foundation.electrical.electrical\"},{\"id\":\"nB\",\"label\":\"B-\",\"type\":\"foundation.electrical.electrical\"}],\"Right\":[{\"id\":\"R\",\"label\":\"R\",\"type\":\"foundation.mechanical.rotational.rotational\"},{\"id\":\"C\",\"label\":\"C\",\"type\":\"foundation.mechanical.rotational.rotational\"}],\"Top\":[]}"
  Stepper Motor Driver : ee_lib/Electromechanical/Reluctance & Stepper/Stepper Motor Driver  Commented=on  step_or_av=1  step_rate_per_volt=1 Hz/V  Venable=2.5 V  Vreverse=2.5 V  supply_ports=ee.enum.supply_ports.hidesupply  Vm=Vdc V  Vsupply=Vdc V  half_stepping=0  stepping_mode=ee.enum.electromech.steppingMode.fullStep  numMicroSteps=2  Im=1 A
      settings: InternalSimscapePortConfiguration="{\"Bottom\":[],\"Left\":[{\"id\":\"ENA\",\"label\":\"ENA\",\"type\":\"foundation.electrical.electrical\"},{\"id\":\"REF\",\"label\":\"REF\",\"type\":\"foundation.electrical.electrical\"},{\"id\":\"REV\",\"label\":\"REV\",\"type\":\"foundation.electrical.electrical\"}],\"Right\":[{\"id\":\"pA\",\"label\":\"A+\",\"type\":\"foundation.electrical.electrical\"},{\"id\":\"nA\",\"label\":\"A-\",\"type\":\"foundation.electrical.electrical\"},{\"id\":\"pB\",\"label\":\"B+\",\"type\":\"foundation.electrical.electrical\"},{\"id\":\"nB\",\"label\":\"B-\",\"type\":\"foundation.electrical.electrical\"}],\"Top\":[]}"
  Subsystem1 : Subsystem  Commented=on
  Sum : Sum  Commented=on  Inputs=|++
  Sum{1..2,5..6,13..14} (6 alike) : Sum  Inputs=|++
  Sum3 : Sum  Commented=on  Inputs=|++
  Sum7 : Sum  Inputs=|+-
  Sum8 : Sum  Inputs=|+-
  Te : Scope  NumInputPorts=3
  Terminator : Terminator  Commented=on
  Terminator1 : Terminator
  Terminator2 : Terminator
  Terminator3 : Terminator
  Theta_e : Scope  NumInputPorts=4
  To Workspace : ToWorkspace  Commented=on  VariableName=Wm_planta_M1  SaveFormat=Timeseries  SampleTime=-1
  To Workspace1 : ToWorkspace  Commented=on  VariableName=Te_planta_M1  SaveFormat=Timeseries  SampleTime=-1
  To Workspace10 : ToWorkspace  VariableName=Ib_planta_M2  SaveFormat=Timeseries  SampleTime=-1
  To Workspace11 : ToWorkspace  VariableName=Ia_planta_M2  SaveFormat=Timeseries  SampleTime=-1
  To Workspace12 : ToWorkspace  VariableName=Wm_planta_M2  SaveFormat=Timeseries  SampleTime=-1
  To Workspace13 : ToWorkspace  VariableName=We_planta_M2  SaveFormat=Timeseries  SampleTime=-1
  To Workspace14 : ToWorkspace  VariableName=theta_e_obs_M2  SaveFormat=Timeseries  SampleTime=-1
  To Workspace15 : ToWorkspace  Commented=on  VariableName=Wm_planta_M0  SaveFormat=Timeseries  SampleTime=-1
  To Workspace16 : ToWorkspace  Commented=on  VariableName=Te_planta_M0  SaveFormat=Timeseries  SampleTime=-1
  To Workspace17 : ToWorkspace  Commented=on  VariableName=Vb_planta_M0  SaveFormat=Timeseries  SampleTime=-1
  To Workspace18 : ToWorkspace  Commented=on  VariableName=Va_planta_M0  SaveFormat=Timeseries  SampleTime=-1
  To Workspace19 : ToWorkspace  Commented=on  VariableName=Ib_planta_M0  SaveFormat=Timeseries  SampleTime=-1
  To Workspace2 : ToWorkspace  Commented=on  VariableName=Vb_planta_M1  SaveFormat=Timeseries  SampleTime=-1
  To Workspace20 : ToWorkspace  Commented=on  VariableName=Ia_planta_M0  SaveFormat=Timeseries  SampleTime=-1
  To Workspace21 : ToWorkspace  Commented=on  VariableName=We_planta_M0  SaveFormat=Timeseries  SampleTime=-1
  To Workspace22 : ToWorkspace  VariableName=Wm_obs_M2  SaveFormat=Timeseries  SampleTime=-1
  To Workspace23 : ToWorkspace  VariableName=theta_e_planta_M2  SaveFormat=Timeseries  SampleTime=-1
  To Workspace24 : ToWorkspace  VariableName=err_theta_deg  SaveFormat=Timeseries  SampleTime=-1
  To Workspace25 : ToWorkspace  VariableName=err_Wm  SaveFormat=Timeseries  SampleTime=-1
  To Workspace26 : ToWorkspace  VariableName=Iq_planta_M1  SaveFormat=Timeseries  SampleTime=-1
  To Workspace27 : ToWorkspace  VariableName=Id_planta_M1  SaveFormat=Timeseries  SampleTime=-1
  To Workspace28 : ToWorkspace  VariableName=Wm_planta_M1  SaveFormat=Timeseries  SampleTime=-1
  To Workspace29 : ToWorkspace  VariableName=We_planta_M1  SaveFormat=Timeseries  SampleTime=-1
  To Workspace3 : ToWorkspace  Commented=on  VariableName=Va_planta_M1  SaveFormat=Timeseries  SampleTime=-1
  To Workspace30 : ToWorkspace  VariableName=theta_e_planta_M  SaveFormat=Timeseries  SampleTime=-1
  To Workspace31 : ToWorkspace  VariableName=Te_planta_M1  SaveFormat=Timeseries  SampleTime=-1
  To Workspace32 : ToWorkspace  VariableName=Vq_planta_M1  SaveFormat=Timeseries  SampleTime=-1
  To Workspace33 : ToWorkspace  VariableName=Vd_planta_M1  SaveFormat=Timeseries  SampleTime=-1
  To Workspace4 : ToWorkspace  Commented=on  VariableName=Ib_planta_M1  SaveFormat=Timeseries  SampleTime=-1
  To Workspace5 : ToWorkspace  Commented=on  VariableName=Ia_planta_M1  SaveFormat=Timeseries  SampleTime=-1
  To Workspace6 : ToWorkspace  Commented=on  VariableName=We_planta_M1  SaveFormat=Timeseries  SampleTime=-1
  To Workspace7 : ToWorkspace  VariableName=Te_planta_M2  SaveFormat=Timeseries  SampleTime=-1
  To Workspace8 : ToWorkspace  VariableName=Vb_planta_M2  SaveFormat=Timeseries  SampleTime=-1
  To Workspace9 : ToWorkspace  VariableName=Va_planta_M2  SaveFormat=Timeseries  SampleTime=-1
  Triangle Generator1 : spsTriangleGeneratorLib/Triangle Generator  Freq=f_carrier  Phase=0  Ts=sample_time
  Triggered Subsystem : Subsystem  Commented=on  TreatAsAtomicUnit=on
  Triggered Subsystem1 : Subsystem  TreatAsAtomicUnit=on  DataTypeOverride=Single
  Triggered Subsystem10 : Subsystem  TreatAsAtomicUnit=on
  Triggered Subsystem2 : Subsystem  Commented=on  TreatAsAtomicUnit=on  DataTypeOverride=Single
  Triggered Subsystem3 : Subsystem  Commented=on  TreatAsAtomicUnit=on  DataTypeOverride=Single
  Triggered Subsystem4 : Subsystem  Commented=on  TreatAsAtomicUnit=on  DataTypeOverride=Single
  Triggered Subsystem5 : Subsystem  TreatAsAtomicUnit=on
  Triggered Subsystem6 : Subsystem  TreatAsAtomicUnit=on
  Triggered Subsystem7 : Subsystem  Commented=on  TreatAsAtomicUnit=on
  Triggered Subsystem8 : Subsystem  Commented=on  TreatAsAtomicUnit=on
  Triggered Subsystem9 : Subsystem  TreatAsAtomicUnit=on
  Unit Delay{1..7,9..10,15,17..26,28..31} (24 alike) : UnitDelay  SampleTime=-1  HasFrameUpgradeWarning=on
  Unit Delay{8,11..14,16,27} (7 alike) : UnitDelay  Commented=on  SampleTime=-1  HasFrameUpgradeWarning=on
  Vab : Scope  NumInputPorts=6
  Valpha_betha : Scope  NumInputPorts=4
  Variable Pulse Generator : VariablePulseGenerator  Commented=on  RunAtFixedTimeIntervals=on  SampleTime=1/frecuency_simulation
  Vdq : Scope  NumInputPorts=4
  Vmag : Scope  NumInputPorts=3
  Voltage Measurement{1..4} (4 alike) : spsVoltageMeasurementLib/Voltage Measurement  Commented=on  PhasorSimulation=off  OutputType=Complex  PSBequivalent=0
  Voltage Sensor : fl_lib/Electrical/Electrical Sensors/Voltage Sensor  Commented=on
  Voltage Sensor1 : fl_lib/Electrical/Electrical Sensors/Voltage Sensor  Commented=on
  Voltage Sensor2 : fl_lib/Electrical/Electrical Sensors/Voltage Sensor  Commented=on
  We : Scope  NumInputPorts=3
  Wm_ref : FromWorkspace  VariableName=Wm_ref  Interpolate=off  OutputAfterFinalValue=Holding final value
  deg : nesl_utility/PS-Simulink Converter  Commented=on  PhysicalDomain=network_engine_domain  SubClassName=ps_output  LeftPortType=input  RightPortType=output  PseudoPeriodic=off  Frequencies=[]  VectorFormat=1-D array  Unit=deg  AffineConversion=off
  deg2 : nesl_utility/PS-Simulink Converter  Commented=on  PhysicalDomain=network_engine_domain  SubClassName=ps_output  LeftPortType=input  RightPortType=output  PseudoPeriodic=off  Frequencies=[]  VectorFormat=1-D array  Unit=rad  AffineConversion=off
  ekf_4var : Demux  Commented=on
  ekf_4var1 : Demux
  powergui : spspowerguiLib/powergui  Priority=1  SimulationMode=Discrete  SampleTime=1/frecuency_simulation  frequency=60  Iterations=50  frequencyindice=0  Pbase=100e6  ErrMax=1e-4  UnitsV=kV  UnitsW=MW  buscounter=0  FunctionMessages=off  echomessages=off  EnableUseOfTLC=off  CurrentSourceSwitches=off  DisableSnubberDevices=off  DisableRonSwitches=off  DisableVfSwitches=off  DisplayEquations=off  AutomaticDiscreteSolvers=off  SolverType=Tustin/Backward Euler (TBE)  Interpol=off  ExternalGateDelay=off  methode=off  Ts=100  x0status=blocks  SPID=on  SwTol=0  HookPort=off  NonlinearTolerance=1e-4  nMaxIteration=100  ContinueOnMaxIteration=off  RestoreLinks=warning  ResistiveCurrentMeasurement=off  Frange=[0:2:500]  Ylog=off  Xlog=on  ShowGrid=off  save=off  variable=ZData  structure=0  ZoomFFT=off  StartTime=0.0  cycles=1  DisplayStyle=1  fundamental=60  FreqAxis=off  MaxFrequency=1000  frequencyindicesteady=1  RmsSteady=1  display=off
  rpm : nesl_utility/PS-Simulink Converter  Commented=on  PhysicalDomain=network_engine_domain  SubClassName=ps_output  LeftPortType=input  RightPortType=output  PseudoPeriodic=off  Frequencies=[]  VectorFormat=1-D array  Unit=rad/s  AffineConversion=off
  rpm1 : nesl_utility/PS-Simulink Converter  Commented=on  PhysicalDomain=network_engine_domain  SubClassName=ps_output  LeftPortType=input  RightPortType=output  PseudoPeriodic=off  Frequencies=[]  VectorFormat=1-D array  Unit=N*m  AffineConversion=off
  rpm2 : nesl_utility/PS-Simulink Converter  Commented=on  PhysicalDomain=network_engine_domain  SubClassName=ps_output  LeftPortType=input  RightPortType=output  PseudoPeriodic=off  Frequencies=[]  VectorFormat=1-D array  Unit=N*m  AffineConversion=off
  tag scope: Iq_ref_M1=global, Iq_ref_M2=global, Te_planta_M1=global, Te_planta_M2=global, We_planta_M1=global, We_planta_M2=global, Wm_planta_M1=global, Wm_planta_M2=global, theta_e_planta_M1=global, theta_e_planta_M2=global
  wires:
  [Te_planta_M1] -> Te/1
  [We_planta_M1] -> We/2
  [Vd_M1] -> Vdq/1
  [Vb_M0] -> Vab/2
  [Iq_M1] -> Idq/2
  [Id_M1] -> Idq/1
  [Va_M0] -> Vab/1
  [Ia_M0] -> Iab/1
  [Ib_M0] -> Iab/2
  [Vq_M1] -> Vdq/2
  [Ia_M1] -> Mux2/1
  [Ib_M1] -> Mux2/2
  Constant11/1 -> Mux2/3
  Mux2/1 -> Clarke to Park Angle Transform1/1
  Clarke to Park Angle Transform1/1 -> Demux2/1
  Demux2/3 -> Terminator1/1
  [Iq_M1] -> Iq/1
  [Iq_ref_M1] -> Iq/2
  [Iq_M1] -> Product/2, Product/1
  [Id_M1] -> Product1/2, Product1/1
  Product/1 -> Sum13/1
  Product1/1 -> Sum13/2
  Sum13/1 -> Sqrt/1
  Sqrt/1 -> Imag/1
  Product3/1 -> Sum14/2
  Sum14/1 -> Sqrt1/1
  [Vq_M1] -> Product2/2, Product2/1
  [Vd_M1] -> Product3/2, Product3/1
  Sqrt1/1 -> Vmag/2
  Product2/1 -> Sum14/1
  Function-Call Generator/1 -> Triggered Subsystem1/Trigger
  [Te_planta_M2] -> Te/2
  [theta_m_planta_M1] -> Scope5/1
  [theta_m_planta_M2] -> Scope5/2
  [Ia_M2] -> Scope6/2
  [Ia_M1] -> Scope6/1
  [Ib_M1] -> Scope12/1
  [Ib_M2] -> Scope12/2
  [Valpha_M1] -> Valpha_betha/1
  [Vbetha_M1] -> Valpha_betha/2
  Gain7/1 -> Goto42/1
  ekf_4var/4 -> MATLAB Function2/1(u)
  ekf_4var/1 -> Goto28/1
  ekf_4var/2 -> Goto29/1
  From19/1 -> ekf_4var/1
  MATLAB Function2/1(y) -> Gain7/1, Goto31/1
  [Valpha_M2] -> Triggered Subsystem1/1(Va)
  [Vbetha_M2] -> Triggered Subsystem1/2(Vb)
  Constant1/1 -> Vmag/1
  Mux/1 -> Goto48/1
  Gain14/1 -> Goto60/1
  Demux3/7 -> MATLAB Function6/1(u)
  Relational Operator6/1 -> Goto63/1, NOT6/1
  From116/1 -> Mosfet13/1
  Relational Operator3/1 -> Goto73/1, NOT3/1
  From111/1 -> Mosfet11/1
  From97/1 -> Mosfet15/1
  Voltage Measurement2/1 -> Mux/1, Simulink-PS Converter1/1, Goto78/1
  PS-Simulink Converter4/1 -> Mux/3, Goto56/1
  Gain9/1 -> Relational Operator6/1, Relational Operator2/1
  Relational Operator2/1 -> NOT2/1, Goto26/1
  MATLAB Function6/1(y) -> Gain14/1, Goto61/1
  NOT3/1 -> Goto75/1
  Demux3/6 -> To Workspace/1, Goto58/1, Gain15/1
  Relational Operator7/1 -> Goto76/1, NOT7/1
  From104/1 -> Mosfet8/1
  Demux3/3 -> To Workspace5/1
  Demux3/4 -> To Workspace4/1
  Demux3/1 -> To Workspace3/1
  From117/1 -> Mosfet14/1
  From109/1 -> Mosfet10/1
  Demux3/5 -> To Workspace1/1, Goto62/1
  NOT2/1 -> Goto32/1
  From115/1 -> Mosfet12/1
  From107/1 -> Mosfet9/1
  Gain13/1 -> Relational Operator7/1, Relational Operator3/1
  NOT6/1 -> Goto70/1
  NOT7/1 -> Goto77/1
  Gain15/1 -> To Workspace6/1, Goto59/1
  From89/1 -> Demux3/1
  From118/1 -> Relational Operator7/2, Relational Operator3/2, Relational Operator2/2, Relational Operator6/2
  [Vb_M1] -> Vab/4
  [Va_M1] -> Vab/3
  [Valpha_M2] -> Valpha_betha/3
  [Vbetha_M2] -> Valpha_betha/4
  [Ib_M1] -> Iab/4
  [Ia_M1] -> Iab/3
  [Vd_M2] -> Vdq/3
  [Vq_M2] -> Vdq/4
  [Id_M2] -> Idq/3
  [Iq_M2] -> Idq/4
  [Iq_M2] -> Iq/4
  [Iq_ref_M2] -> Iq/5
  Product4/1 -> Sum1/1
  [Id_M2] -> Product5/2, Product5/1
  Sum1/1 -> Sqrt2/1
  [Iq_M2] -> Product4/2, Product4/1
  Product5/1 -> Sum1/2
  Product7/1 -> Sum2/2
  [Vq_M2] -> Product6/2, Product6/1
  Sum2/1 -> Sqrt3/1
  [Vd_M2] -> Product7/2, Product7/1
  Product6/1 -> Sum2/1
  Sqrt3/1 -> Vmag/3
  Triangle Generator1/1 -> [carrier]
  ekf_4var/3 -> Goto30/1
  Function-Call Generator2/1 -> Triggered Subsystem3/Trigger
  Gain5/1 -> Goto45/1
  Triggered Subsystem3/3(Tx_hat) -> Goto35/1
  Triggered Subsystem3/2(We_hat) -> Gain5/1, Goto34/1
  From24/1 -> Triggered Subsystem3/2(Iq_obs)
  NOT8/1 -> Goto33/1
  From48/1 -> Mosfet5/1
  Relational Operator1/1 -> NOT1/1, Goto1/1
  From59/1 -> Relational Operator8/2, Relational Operator4/2, Relational Operator1/2, Relational Operator5/2
  From62/1 -> Mosfet6/1
  MATLAB Function3/1(y) -> [theta_m_planta_M2]
  Gain1/1 -> Relational Operator4/1, Relational Operator8/1
  Gain8/1 -> Relational Operator5/1, Relational Operator1/1
  From39/1 -> Mosfet3/1
  From7/1 -> Mosfet16/1
  Relational Operator4/1 -> Goto22/1, NOT4/1
  NOT4/1 -> Goto23/1
  Relational Operator5/1 -> Goto13/1, NOT5/1
  MATLAB Function4/1(y) -> To Workspace23/1, [theta_e_planta_M2]
  From4/1 -> Mosfet7/1
  NOT5/1 -> Goto18/1
  NOT1/1 -> Goto2/1
  From40/1 -> Mosfet4/1
  From11/1 -> Mosfet2/1
  Relational Operator8/1 -> Goto25/1, NOT8/1
  From9/1 -> Mosfet1/1
  [Wm_ref] -> Scope2/1
  Function-Call Generator4/1 -> Triggered Subsystem5/Trigger
  Function-Call Generator5/1 -> Triggered Subsystem6/Trigger
  [Wm_ref] -> Triggered Subsystem6/1(Wm_ref)
  Triggered Subsystem5/1(Vd) -> [Vd_M2]
  Triggered Subsystem5/2(Vq) -> [Vq_M2]
  Triggered Subsystem5/3(Id) -> [Id_M2]
  Triggered Subsystem5/4(Iq) -> [Iq_M2]
  [We_planta_M2] -> We/3
  Demux3/2 -> To Workspace2/1
  [var_stepper_M2] -> Demux/1
  Demux/1 -> To Workspace9/1
  Demux/2 -> To Workspace8/1
  Demux/3 -> To Workspace11/1, [Ia_M2]
  Demux/4 -> To Workspace10/1, [Ib_M2]
  From88/1 -> Triggered Subsystem8/2(Wm)
  From85/1 -> Triggered Subsystem7/3(Wm)
  Triggered Subsystem7/1(Vd) -> Goto50/1
  From86/1 -> Triggered Subsystem7/2(Ib)
  From90/1 -> Triggered Subsystem7/1(Ia)
  Triggered Subsystem7/4(Iq) -> Goto80/1
  Triggered Subsystem7/3(Id) -> Goto67/1
  Triggered Subsystem7/2(Vq) -> Goto54/1
  From87/1 -> Triggered Subsystem7/4(Theta)
  Function-Call Generator7/1 -> Triggered Subsystem8/Trigger
  From92/1 -> Triggered Subsystem8/3(Tl_Tdm)
  Triggered Subsystem8/1(Iq_ref) -> Goto69/1
  From91/1 -> Triggered Subsystem7/5(Iq_ref)
  From65/1 -> Triggered Subsystem8/1(Wm_ref)
  Function-Call Generator6/1 -> Triggered Subsystem7/Trigger
  MATLAB Function5/1(y) -> Gain11/1, Goto91/1
  Gain12/1 -> To Workspace21/1, Goto89/1
  Gain11/1 -> Goto90/1
  [We_planta_M0] -> We/1
  Meas 1/1(SL) -> ENA or step rate/1
  Constant4/1 -> Variable Pulse Generator/1
  Divide/1 -> Variable Pulse Generator/2
  Constant5/1 -> Divide/1
  Gain/1 -> Divide/2
  From/1 -> Gain/1
  Variable Pulse Generator/1 -> Gain10/1
  Gain10/1 -> Simulink-PS Converter/1
  1/step angle/1 -> Results/1
  deg/1 -> 1/step angle/1
  deg2/1 -> MATLAB Function5/1(u), Results/2
  rpm/1 -> To Workspace15/1, Goto88/1, Gain12/1
  rpm1/1 -> Scope/1
  rpm2/1 -> Scope24/1
  PS-Simulink Converter5/1 -> Mux/4, Goto57/1
  Gain17/1 -> Mux/5
  Voltage Measurement3/1 -> Mux/2, Goto79/1, Simulink-PS Converter2/1
  PS-Simulink Converter6/1 -> Scope1/1, Mux/6
  PS-Simulink Converter7/1 -> Mux/7
  From38/1 -> Cos/1, Sin/1
  Sin/1 -> Product8/1
  From63/1 -> Product8/2
  Cos/1 -> Product9/1
  From93/1 -> Product9/2
  Product8/1 -> Sum/1
  Product9/1 -> Sum/2
  Sum/1 -> Gain17/1
  Product10/1 -> Sum3/1
  Cos1/1 -> Product11/1
  From94/1 -> Cos1/1, Sin1/1
  From96/1 -> Product11/2
  Product11/1 -> Sum3/2
  Sum3/1 -> Gain18/1
  Sin1/1 -> Product10/1
  From95/1 -> Product10/2
  PS-Simulink Converter2/1 -> Goto4/1
  PS-Simulink Converter3/1 -> Goto14/1
  PS-Simulink Converter/1 -> Goto16/1
  PS-Simulink Converter1/1 -> Goto15/1
  Gain18/1 -> Goto92/1, To Workspace16/1
  From110/1 -> To Workspace19/1
  From112/1 -> To Workspace20/1
  From103/1 -> To Workspace17/1
  From98/1 -> To Workspace18/1
  [Va_M2] -> Vab/6
  [Vb_M2] -> Vab/5
  [Ia_M2] -> Iab/5
  [Ib_M2] -> Iab/6
  ekf_4var1/2 -> [Iq_obs_M2]
  [x_ekf_4var_M2] -> ekf_4var1/1
  ekf_4var1/3 -> To Workspace22/1, [Wm_obs_M2]
  ekf_4var1/4 -> MATLAB Function1/1(u)
  ekf_4var1/1 -> [Id_obs_M2]
  MATLAB Function1/1(y) -> Gain4/1, Scope4/1, [theta_m_obs_M2]
  [Tx_hat_M2] -> Gain20/1
  [Ia_obs_M2] -> Scope6/3
  [Ib_obs_M2] -> Scope12/3
  Triggered Subsystem3/1(Theta_e_hat) -> Goto44/1
  [Id_M1] -> Id/1
  [Id_M2] -> Id/3
  [Ib_M2] -> Mux5/2
  Mux5/1 -> Clarke to Park Angle Transform/1
  [Ia_M2] -> Mux5/1
  Constant6/1 -> Mux5/3
  Clarke to Park Angle Transform/1 -> Demux1/1
  Demux1/3 -> Terminator2/1
  Demux2/1 -> [Id_real_M1]
  Demux2/2 -> [Iq_real_M1]
  Demux1/1 -> [Id_real_M2]
  Demux1/2 -> [Iq_real_M2]
  [Iq_M1] -> Iq/3
  [Iq_real_M2] -> Iq/6
  [Id_M1] -> Id/2
  [Id_real_M2] -> Id/4
  Product15/1 -> Sum5/2
  [Id_real_M1] -> Product15/2, Product15/1
  [Iq_real_M1] -> Product14/2, Product14/1
  Sum5/1 -> Sqrt4/1
  Product14/1 -> Sum5/1
  Sum6/1 -> Sqrt5/1
  [Id_real_M2] -> Product17/2, Product17/1
  [Iq_real_M2] -> Product16/2, Product16/1
  Product17/1 -> Sum6/2
  Product16/1 -> Sum6/1
  Sqrt4/1 -> Imag/2
  Sqrt5/1 -> Imag/4
  Sqrt2/1 -> Imag/3
  Constant10/1 -> Mux1/3
  Mux1/1 -> Park to Clarke Angle Transform1/1
  From105/1 -> Mux1/1
  From106/1 -> Mux1/2
  From108/1 -> Park to Clarke Angle Transform1/2
  Demux4/1 -> Unit Delay13/1, Gain9/1
  Demux4/2 -> Gain13/1, Unit Delay14/1
  Demux4/3 -> Terminator/1
  Unit Delay13/1 -> Goto71/1
  Unit Delay14/1 -> Goto72/1
  Gain4/1 -> To Workspace14/1, [theta_e_obs_M2]
  [theta_e_hat_M2] -> MATLAB Function14/1(u)
  [theta_e_obs_M2] -> MATLAB Function12/1(u)
  [theta_e_planta_M2] -> MATLAB Function10/1(u)
  [theta_e_planta_M1] -> MATLAB Function9/1(u)
  [theta_e_planta_M2] -> Sum8/1
  [theta_e_obs_M2] -> Sum8/2
  Sum8/1 -> Cos3/1, Sin3/1
  Atan2/1 -> Gain21/1
  Gain21/1 -> To Workspace24/1, Scope14/1
  Voltage Measurement4/1 -> Goto51/1
  MATLAB Function10/1(y) -> Gain26/1
  MATLAB Function14/1(y) -> Gain30/1
  MATLAB Function12/1(y) -> Gain28/1
  MATLAB Function9/1(y) -> Gain25/1
  Gain25/1 -> Theta_e/1
  Gain26/1 -> Theta_e/2
  Gain28/1 -> Theta_e/3
  Gain30/1 -> Theta_e/4
  Unit Delay4/1 -> Clarke to Park Angle Transform/2
  [theta_e_planta_M2] -> Unit Delay4/1
  [theta_e_planta_M1] -> Unit Delay18/1
  Unit Delay18/1 -> Clarke to Park Angle Transform1/2
  Sin3/1 -> Atan2/1
  Cos3/1 -> Atan2/2
  [Wm_obs_M2] -> Sum7/2
  [Wm_planta_M2] -> Sum7/1
  Sum7/1 -> To Workspace25/1, Scope15/1
  Voltage Measurement1/1 -> Goto17/1
  Constant8/1 -> Level-2 MATLAB S-Function/3
  Level-2 MATLAB S-Function/1 -> Mux4/3
  Level-2 MATLAB S-Function/2 -> Mux4/4
  Mux4/1 -> [var_stepper_M2]
  Park to Clarke Angle Transform1/1 -> Demux4/1
  Level-2 MATLAB S-Function/3 -> Mux4/5
  Level-2 MATLAB S-Function/4 -> Mux4/6
  Level-2 MATLAB S-Function/5 -> Mux4/7
  Level-2 MATLAB S-Function/6 -> Mux4/8
  Level-2 MATLAB S-Function/7 -> Mux4/9
  Demux/5 -> To Workspace12/1, [Wm_planta_M2]
  Demux/6 -> To Workspace13/1, [We_planta_M2]
  Demux/7 -> MATLAB Function3/1(u)
  Demux/8 -> MATLAB Function4/1(u)
  Demux/9 -> To Workspace7/1, [Te_planta_M2]
  Triggered Subsystem5/6(Vbetha) -> [Vbetha_M2]
  Triggered Subsystem5/5(Valpha) -> [Valpha_M2]
  [Iq_ref_M2] -> Triggered Subsystem5/5(Iq_ref)
  Triggered Subsystem6/1(Iq_ref) -> [Iq_ref_M2]
  [Wm_planta_M1] -> Scope2/2
  [Wm_planta_M2] -> Scope2/3
  [Wm_obs_M2] -> Scope2/4
  [Wm_hat_M2] -> Scope2/5
  Triggered Subsystem1/1(kf_4var2) -> [x_ekf_4var_M2]
  [Id_obs_M2] -> Mux3/1
  Mux3/1 -> Park to Clarke Angle Transform/1
  Constant2/1 -> Mux3/3
  [Iq_obs_M2] -> Mux3/2
  [theta_e_planta_M2] -> Unit Delay7/1
  Unit Delay7/1 -> Park to Clarke Angle Transform/2
  Demux5/2 -> [Ib_obs_M2]
  Demux5/1 -> [Ia_obs_M2]
  Demux5/3 -> Terminator3/1
  Park to Clarke Angle Transform/1 -> Demux5/1
  Triggered Subsystem2/1(kf_4var2) -> Unit Delay16/1
  Demux6/3 -> To Workspace27/1, [Id_M1]
  From131/1 -> Triggered Subsystem2/4(Ib)
  Level-2 MATLAB S-Function1/3 -> Mux6/5
  Level-2 MATLAB S-Function1/2 -> Mux6/4
  Demux6/6 -> To Workspace29/1, [We_planta_M1]
  Demux6/4 -> To Workspace26/1, [Iq_M1]
  Demux6/8 -> MATLAB Function11/1(u)
  From132/1 -> Triggered Subsystem4/2(Iq_obs)
  Function-Call Generator8/1 -> Triggered Subsystem9/Trigger
  Triggered Subsystem4/3(Tx_hat) -> Unit Delay11/1
  Level-2 MATLAB S-Function1/5 -> Mux6/7
  Unit Delay12/1 -> Gain3/1, Goto100/1
  From159/1 -> Triggered Subsystem4/1(theta_e)
  Function-Call Generator1/1 -> Triggered Subsystem2/Trigger
  [var_stepper_M1] -> Demux6/1
  Triggered Subsystem10/2(Wm_filt_out) -> [Wm_filt_M1]
  Triggered Subsystem9/3(Valpha) -> [Valpha_M1]
  Demux6/2 -> To Workspace32/1
  Triggered Subsystem4/1(Theta_e_hat) -> Unit Delay8/1
  Level-2 MATLAB S-Function1/6 -> Mux6/8
  Demux6/9 -> To Workspace31/1, [Te_planta_M1]
  MATLAB Function11/1(y) -> To Workspace30/1, [theta_e_planta_M1]
  Demux6/1 -> To Workspace33/1
  Unit Delay16/1 -> Goto97/1
  Demux6/5 -> To Workspace28/1, [Wm_planta_M1]
  Triggered Subsystem9/4(Vbetha) -> [Vbetha_M1]
  Mux6/1 -> [var_stepper_M1]
  MATLAB Function8/1(y) -> [theta_m_planta_M1]
  Demux6/7 -> MATLAB Function8/1(u)
  Level-2 MATLAB S-Function1/7 -> Mux6/9
  Constant7/1 -> Level-2 MATLAB S-Function1/3
  Triggered Subsystem4/2(We_hat) -> Unit Delay12/1
  Level-2 MATLAB S-Function1/4 -> Mux6/6
  Triggered Subsystem10/1(Iq_ref) -> [Iq_ref_M1]
  From136/1 -> Triggered Subsystem2/5(Theta_e)
  From128/1 -> Triggered Subsystem2/1(Va)
  Gain3/1 -> Goto105/1
  From130/1 -> Triggered Subsystem2/3(Ia)
  Level-2 MATLAB S-Function1/1 -> Mux6/3
  From129/1 -> Triggered Subsystem2/2(Vb)
  Unit Delay11/1 -> Goto101/1
  [Wm_ref] -> Triggered Subsystem10/1(Wm_ref)
  Unit Delay8/1 -> Goto104/1
  Function-Call Generator9/1 -> Triggered Subsystem10/Trigger
  [Iq_ref_M1] -> Triggered Subsystem9/5(Iq_ref)
  Function-Call Generator3/1 -> Triggered Subsystem4/Trigger
  Triggered Subsystem9/1(Vd) -> [Vd_M1]
  Triggered Subsystem9/2(Vq) -> [Vq_M1]
  [Vbetha_M2] -> Unit Delay5/1
  Unit Delay5/1 -> Level-2 MATLAB S-Function/2, Mux4/2
  [Valpha_M2] -> Unit Delay10/1
  Unit Delay10/1 -> Mux4/1, Level-2 MATLAB S-Function/1
  [Vq_M1] -> Unit Delay17/1
  [Vd_M1] -> Unit Delay15/1
  Unit Delay15/1 -> Level-2 MATLAB S-Function1/1, Mux6/1
  Unit Delay17/1 -> Mux6/2, Level-2 MATLAB S-Function1/2
  [Wm_planta_M1] -> Unit Delay19/1
  Unit Delay19/1 -> Triggered Subsystem10/2(Wm)
  [theta_e_planta_M1] -> Unit Delay20/1
  Unit Delay20/1 -> Triggered Subsystem10/4(theta_e)
  Unit Delay24/1 -> Triggered Subsystem9/4(Theta)
  [theta_e_planta_M1] -> Unit Delay24/1
  Unit Delay23/1 -> Triggered Subsystem9/3(Wm)
  [Wm_planta_M1] -> Unit Delay23/1
  Unit Delay22/1 -> Triggered Subsystem9/2(Ib)
  [Iq_M1] -> Unit Delay22/1
  Unit Delay21/1 -> Triggered Subsystem9/1(Ia)
  [Id_M1] -> Unit Delay21/1
  Gain20/1 -> Te/3
  Unit Delay25/1 -> Triggered Subsystem1/4(Ib)
  [Ib_M2] -> Unit Delay25/1
  [Ia_M2] -> Unit Delay9/1
  Unit Delay9/1 -> Triggered Subsystem1/3(Ia)
  [theta_e_planta_M2] -> Unit Delay26/1
  From69/1 -> Unit Delay27/1
  Unit Delay27/1 -> Triggered Subsystem3/1(theta_e)
  Unit Delay1/1 -> Triggered Subsystem5/1(Ia)
  [Ia_M2] -> Unit Delay1/1
  Unit Delay2/1 -> Triggered Subsystem5/2(Ib)
  [Ib_M2] -> Unit Delay2/1
  [theta_e_planta_M2] -> Unit Delay3/1
  Unit Delay3/1 -> Triggered Subsystem5/4(Theta)
  From3/1 -> Triggered Subsystem3/3(Id_obs)
  Triggered Subsystem1/2(d_hat) -> [Tx_hat_M2]
  Unit Delay28/1 -> Triggered Subsystem5/3(Wm)
  [Wm_planta_M2] -> Unit Delay28/1
  Unit Delay29/1 -> Triggered Subsystem6/4(theta_m)
  [theta_m_planta_M2] -> Unit Delay29/1
  [Wm_planta_M2] -> Unit Delay30/1
  Unit Delay30/1 -> Triggered Subsystem6/2(Wm)
  Unit Delay31/1 -> Triggered Subsystem6/3(Tl_Tdm)
  Unit Delay6/1 -> Triggered Subsystem10/3(Tl_Tdm)
  Unit Delay26/1 -> Triggered Subsystem1/5(Theta_e)
  Function-Call Generator10/1 -> ?
  ? -> [Alpha_ref]
  [Alpha_ref] -> Triggered Subsystem6/5(alpha_ref)
  Wm_ref/1 -> [Wm_ref]
  [Tx_hat_M2] -> Unit Delay31/1
  connections:
  Mosfet8/LConn1 -- DC Voltage Source2/RConn1 -- Mosfet9/LConn1
  Voltage Measurement2/LConn1 -- Mosfet10/LConn1 -- Mosfet8/RConn1
  Mosfet15/RConn1 -- Mosfet14/RConn1 -- DC Voltage Source3/LConn1
  Mosfet12/RConn1 -- Voltage Measurement3/LConn1 -- Mosfet14/LConn1
  Mosfet13/RConn1 -- Voltage Measurement3/LConn2 -- Mosfet15/LConn1
  Mosfet12/LConn1 -- DC Voltage Source3/RConn1 -- Mosfet13/LConn1
  Mosfet9/RConn1 -- Voltage Measurement2/LConn2 -- Mosfet11/LConn1
  Mosfet11/RConn1 -- Mosfet10/RConn1 -- DC Voltage Source2/LConn1
  Mosfet5/LConn1 -- Voltage Measurement4/LConn1 -- Mosfet3/RConn1
  Mosfet2/LConn1 -- Voltage Measurement1/LConn2 -- Mosfet16/RConn1
  Mosfet4/LConn1 -- Mosfet3/LConn1 -- DC Voltage Source4/RConn1
  Mosfet6/LConn1 -- Mosfet4/RConn1 -- Voltage Measurement4/LConn2
  DC Voltage Source4/LConn1 -- Mosfet6/RConn1 -- Mosfet5/RConn1
  Mosfet16/LConn1 -- Mosfet7/LConn1 -- DC Voltage Source1/RConn1
  Mosfet1/LConn1 -- Voltage Measurement1/LConn1 -- Mosfet7/RConn1
  DC Voltage Source1/LConn1 -- Mosfet2/RConn1 -- Mosfet1/RConn1
  ERef B-/LConn1 -- Stepper Motor Driver/RConn4 -- Voltage Sensor1/RConn2 -- Stepper Motor/LConn4
  ERef A+/LConn1 -- Voltage Sensor/RConn2 -- Stepper Motor Driver/RConn2 -- Stepper Motor/LConn2
  Meas 1/LConn1 -- Controlled Voltage Source/LConn1 -- Stepper Motor Driver/LConn1
  Voltage Sensor/LConn1 -- Current Sensor/LConn1 -- Stepper Motor Driver/RConn1
  Stepper Motor Driver/RConn3 -- Current Sensor1/LConn1 -- Voltage Sensor1/LConn1
  Stepper Motor Driver/LConn3 -- Stepper Motor Driver/LConn2 -- ERef B-1/LConn1 -- Controlled Voltage Source/RConn2
  Voltage Sensor/RConn1 -- PS-Simulink Converter/LConn1
  PS-Simulink Converter1/LConn1 -- Voltage Sensor1/RConn1
  Simulink-PS Converter/RConn1 -- Controlled Voltage Source/RConn1
  Current Sensor/RConn2 -- Stepper Motor/LConn1
  Current Sensor1/RConn2 -- Stepper Motor/LConn3
  Current Sensor/RConn1 -- PS-Simulink Converter2/LConn1
  Current Sensor1/RConn1 -- PS-Simulink Converter3/LConn1
  MRRef Motor/LConn1 -- Rotational Friction3/RConn1 -- Ideal Rotational Motion Sensor/RConn1 -- Solver Configuration/RConn1 -- Stepper Motor/RConn2
  Ideal Torque Sensor/RConn1 -- Rotational Friction3/LConn1 -- Ideal Rotational Motion Sensor/LConn1 -- Inertia/LConn1
  Ideal Rotational Motion Sensor/RConn3 -- deg2/LConn1 -- deg/LConn1
  Ideal Rotational Motion Sensor/RConn2 -- rpm/LConn1
  Stepper Motor/RConn1 -- Ideal Torque Sensor/LConn1
  Ideal Torque Sensor/RConn2 -- rpm1/LConn1
  Inertia1/LConn1 -- Rotational Friction1/LConn1 -- Ideal Torque Sensor1/RConn1 -- Ideal Rotational Motion Sensor1/LConn1
  Stepper Motor1/RConn2 -- Rotational Friction1/RConn1 -- Ideal Rotational Motion Sensor1/RConn1 -- MRRef Motor2/LConn1 -- Solver Configuration1/RConn1
  Ideal Torque Sensor1/RConn2 -- rpm2/LConn1
  Stepper Motor1/RConn1 -- Ideal Torque Sensor1/LConn1
  Controlled Voltage Source1/RConn2 -- Voltage Sensor2/RConn2 -- ERef B-3/LConn1 -- Stepper Motor1/LConn2
  Simulink-PS Converter1/RConn1 -- Controlled Voltage Source1/RConn1
  Controlled Voltage Source2/RConn2 -- Stepper Motor1/LConn4 -- ERef B-2/LConn1
  Controlled Voltage Source2/RConn1 -- Simulink-PS Converter2/RConn1
  Controlled Voltage Source1/LConn1 -- Voltage Sensor2/LConn1 -- Current Sensor2/LConn1
  Current Sensor2/RConn2 -- Stepper Motor1/LConn1
  Current Sensor3/RConn2 -- Stepper Motor1/LConn3
  Controlled Voltage Source2/LConn1 -- Current Sensor3/LConn1
  Current Sensor2/RConn1 -- PS-Simulink Converter4/LConn1
  PS-Simulink Converter5/LConn1 -- Current Sensor3/RConn1
  Ideal Rotational Motion Sensor1/RConn2 -- PS-Simulink Converter6/LConn1
  Ideal Rotational Motion Sensor1/RConn3 -- PS-Simulink Converter7/LConn1
